simulink model "full_sys_Harness1"  (R2022a)
settings: Solver=FixedStepAuto  StartTime=0.0  StopTime=10.0  RelTol=1e-3  EnableMultiTasking=on
undefined symbols (not defined in the file): sigbuilder_block
settings Model: Creator=FUGAZI  LastModifiedBy=FUGAZI
settings SolverCC: AutoInsertRateTranBlk=on
settings OptimizationCC: EnhancedBackFolding=on  PassReuseOutputArgsAs=Individual arguments  ZeroExternalMemoryAtStartup=off  ZeroInternalMemoryAtStartup=off  MaxStackSize=64  OptimizeBlockOrder=speed  DifferentSizesBufferReuse=on  OptimizationCustomize=off  EfficientTunableParamExpr=on
settings DebuggingCC: ParameterTunabilityLossMsg=error
settings HardwareCC: ProdBitPerPointer=32  ProdBitPerSizeT=32  ProdBitPerPtrDiffT=32  ProdLargestAtomicInteger=Long  ProdLargestAtomicFloat=Double  ProdWordSize=32  ProdLongLongMode=on  ProdHWDeviceType=ARM Compatible->ARM Cortex
settings SFSimCC: MATLABDynamicMemAlloc=off
settings RTWCC: SystemTargetFile=ert.tlc  HardwareBoard=STM32 Nucleo L476RG  TemplateMakefile=ert_default_tmf  Toolchain=GNU Tools for ARM Embedded Processors
settings CodeAppCC: ForceParamTrailComments=on  IgnoreCustomStorageClasses=off  OperatorAnnotations=on  SimulinkDataObjDesc=on  SFDataObjDesc=on  InsertBlockDesc=on
settings ERTTargetCC: ExtModeTransport=3  ExtModeStaticAlloc=on  ExtModeStaticAllocSize=2000  ExtModeMexFile=ext_xcp  ExtModeIntrfLevel=Level2 - Open

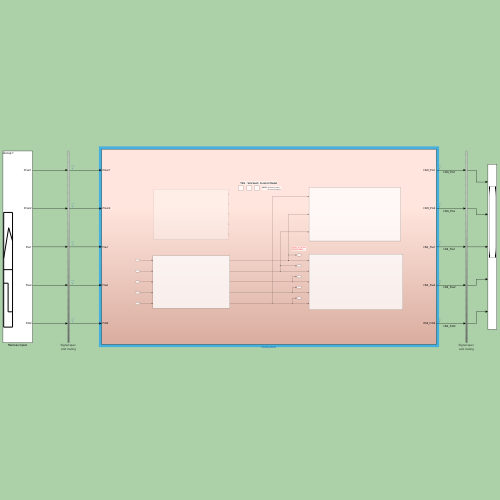
[thumbnail: Simulink's stored preview of the top-level diagram]
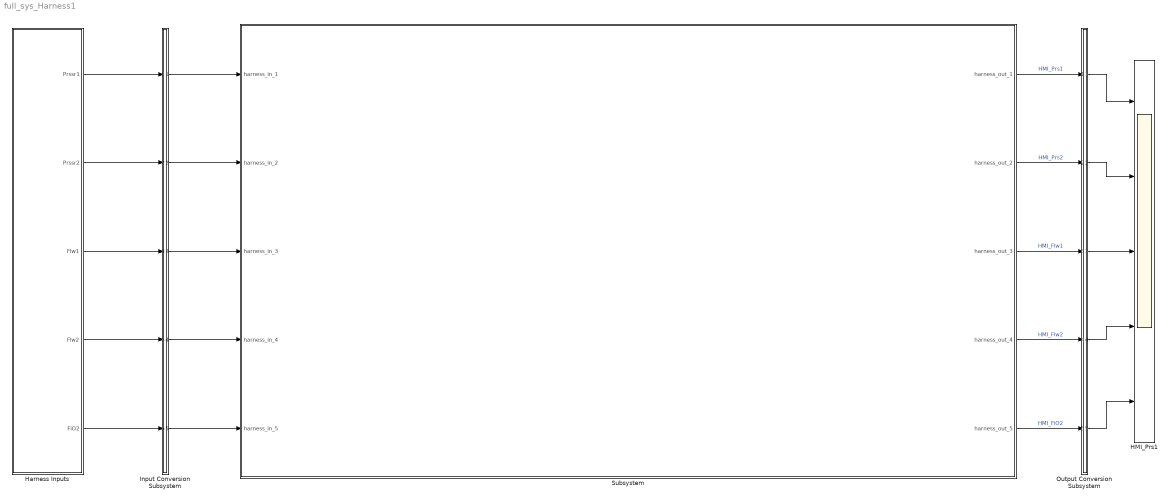
== system full_sys_Harness1 ==
  HMI_Prs1 : Scope
  Harness Inputs : Subsystem  Tag=STV Subsys  LoadFcn=sigbuilder_block('load');  StartFcn=sigbuilder_block('start');  StopFcn=sigbuilder_block('stop');  ClipboardFcn=sigbuilder_block('clipboard');  mask(Sigbuilder block){tuvar=[0:10]}
      mask init:
      | if ~strcmp(get_param(bdroot(gcb),'SimulationStatus'),'stopped'),tuvar = sigbuilder_block('maskInit'); end
      settings: CopyFcn=sigbuilder_block('copy');  DeleteFcn=sigbuilder_block('delete');  ModelCloseFcn=sigbuilder_block('modelClose');  PreSaveFcn=sigbuilder_block('preSave');  PauseFcn=sigbuilder_block('pause');  ContinueFcn=sigbuilder_block('continue');  NameChangeFcn=sigbuilder_block('namechange');  OpenFcn=sigbuilder_block('open',[127.2 33.6 1012.8 503.4 ]);  CloseFcn=sigbuilder_block('close');
      mask Display: plot(0, 0, 100, 100,[2, 2, 32, 32, 2], [68, 8, 8, 68, 68],[32, 2], [38, 38], [32, 19, 2],[53, 60, 44], [32, 17, 17, 2],[16, 16, 31, 31]);txt = getActiveGroup(gcbh);text(2, 100, txt,'verticalAlignment', 'top');
  Input Conversion Subsystem : Subsystem  Tag=__SLT_ICS__  Description=|
      | Signal spec.
      | and routing
      settings: AttributesFormatString=%<Description>
  Output Conversion Subsystem : Subsystem  Tag=__SLT_OCS__  Description=|
      | Signal spec.
      | and routing
      settings: AttributesFormatString=%<Description>
  Subsystem : Subsystem  Tag=__SL_testing_harness_stub_
  wires:
  Harness Inputs/1(Prssr1) -> Input Conversion Subsystem/1(Inport_1)
  Harness Inputs/2(Prssr2) -> Input Conversion Subsystem/2(Inport_2)
  Harness Inputs/3(Flw1) -> Input Conversion Subsystem/3(Inport_3)
  Harness Inputs/4(Flw2) -> Input Conversion Subsystem/4(Inport_4)
  Harness Inputs/5(FiO2) -> Input Conversion Subsystem/5(Inport_5)
  Output Conversion Subsystem/1(Outport_1) -> HMI_Prs1/1
  Output Conversion Subsystem/2(Outport_2) -> HMI_Prs1/2
  Output Conversion Subsystem/3(Outport_3) -> HMI_Prs1/3
  Output Conversion Subsystem/4(Outport_4) -> HMI_Prs1/4
  Output Conversion Subsystem/5(Outport_5) -> HMI_Prs1/5
  Input Conversion Subsystem/1(Outport_1) -> Subsystem/1(harness_in_1)
  Input Conversion Subsystem/2(Outport_2) -> Subsystem/2(harness_in_2)
  Input Conversion Subsystem/3(Outport_3) -> Subsystem/3(harness_in_3)
  Input Conversion Subsystem/4(Outport_4) -> Subsystem/4(harness_in_4)
  Input Conversion Subsystem/5(Outport_5) -> Subsystem/5(harness_in_5)
  Subsystem/1(harness_out_1) -> Output Conversion Subsystem/1(Inport_1)  "HMI_Prs1"
  Subsystem/2(harness_out_2) -> Output Conversion Subsystem/2(Inport_2)  "HMI_Prs2"
  Subsystem/3(harness_out_3) -> Output Conversion Subsystem/3(Inport_3)  "HMI_Flw1"
  Subsystem/4(harness_out_4) -> Output Conversion Subsystem/4(Inport_4)  "HMI_Flw2"
  Subsystem/5(harness_out_5) -> Output Conversion Subsystem/5(Inport_5)  "HMI_FiO2"

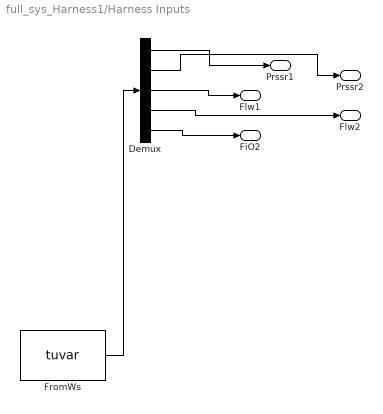
== system full_sys_Harness1/Harness Inputs ==
  Demux : Demux  Tag=STV Demux  Outputs=5
  FromWs : FromWorkspace  Tag=STV FromWs  VariableName=tuvar
      SigBuilderData=|
      | dataSet.timeRange = [0 20]
      | dataSet.name = 'Group 1'
      | sbobj.Name = 'Signal Builder'
      | sbobj.Groups.Name = 'Group 1'
      | sbobj.Groups.Signals(1).Name = 'Prssr1'
      | sbobj.Groups.Signals(1).XData = [0 0.099 2 2 4 4 6 6 8 8 10 10 12 12 14 14 16 16 18 18 20]
      | sbobj.Groups.Signals(1).YData = [0 0 0 6 6 16 16 5 5 18 18 8 8 15 15 4.5 4.5 19 19 0 0]
      | sbobj.Groups.Signals(2).Name = 'Prssr2'
      | sbobj.Groups.Signals(2).XData = [0 2 2 4 4 6 6 7.98 7.98 9.98 9.98 12 12 20]
      | sbobj.Groups.Signals(2).YData = [0 0 5.5 5.5 15 15 6 6 18 18 5 5 0 0]
      | sbobj.Groups.Signals(3).Name = 'Flw1'
      | sbobj.Groups.Signals(3).XData = [0 20]
      | sbobj.Groups.Signals(3).YData = [0 0]
      | sbobj.Groups.Signals(4).Name = 'Flw2'
      | sbobj.Groups.Signals(4).XData = [0 20]
      | sbobj.Groups.Signals(4).YData = [0 0]
      | sbobj.Groups.Signals(5).Name = 'FiO2'
      | sbobj.Groups.Signals(5).XData = [0 20]
      | sbobj.Groups.Signals(5).YData = [0 0]
      | sbobj.Groups.TimeRange = [0 20]
  Prssr1 : Outport  Tag=STV Outport
  Prssr2 : Outport  Tag=STV Outport  Port=2
  Flw1 : Outport  Tag=STV Outport  Port=3
  Flw2 : Outport  Tag=STV Outport  Port=4
  FiO2 : Outport  Tag=STV Outport  Port=5
  wires:
  FromWs/1 -> Demux/1
  Demux/1 -> Prssr1/1
  Demux/2 -> Prssr2/1
  Demux/3 -> Flw1/1
  Demux/4 -> Flw2/1
  Demux/5 -> FiO2/1

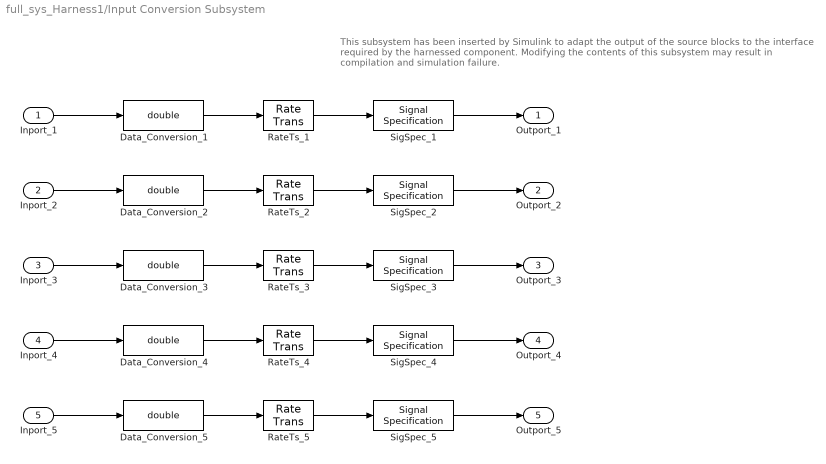
== system full_sys_Harness1/Input Conversion Subsystem ==
  note: This subsystem has been inserted by Simulink to adapt the output of the source blocks to the interface required by the harnessed component.
      |  Modifying the contents of this subsystem may result in compilation and simulation failure.
  Inport_1 : Inport
  Inport_2 : Inport  Port=2
  Inport_3 : Inport  Port=3
  Inport_4 : Inport  Port=4
  Inport_5 : Inport  Port=5
  Data_Conversion_{1..5} (5 alike) : DataTypeConversion  OutDataTypeStr=double
  RateTs_{1..5} (5 alike) : RateTransition  OutPortSampleTime=[-1, 0]
  SigSpec_{1..5} (5 alike) : SignalSpecification  OutDataTypeStr=double  Dimensions=[1]  SampleTime=[-1, 0]
  Outport_1 : Outport
  Outport_2 : Outport  Port=2
  Outport_3 : Outport  Port=3
  Outport_4 : Outport  Port=4
  Outport_5 : Outport  Port=5
  wires:
  SigSpec_1/1 -> Outport_1/1
  RateTs_1/1 -> SigSpec_1/1
  Data_Conversion_1/1 -> RateTs_1/1
  Inport_1/1 -> Data_Conversion_1/1
  SigSpec_2/1 -> Outport_2/1
  RateTs_2/1 -> SigSpec_2/1
  Data_Conversion_2/1 -> RateTs_2/1
  Inport_2/1 -> Data_Conversion_2/1
  SigSpec_3/1 -> Outport_3/1
  RateTs_3/1 -> SigSpec_3/1
  Data_Conversion_3/1 -> RateTs_3/1
  Inport_3/1 -> Data_Conversion_3/1
  SigSpec_4/1 -> Outport_4/1
  RateTs_4/1 -> SigSpec_4/1
  Data_Conversion_4/1 -> RateTs_4/1
  Inport_4/1 -> Data_Conversion_4/1
  SigSpec_5/1 -> Outport_5/1
  RateTs_5/1 -> SigSpec_5/1
  Data_Conversion_5/1 -> RateTs_5/1
  Inport_5/1 -> Data_Conversion_5/1

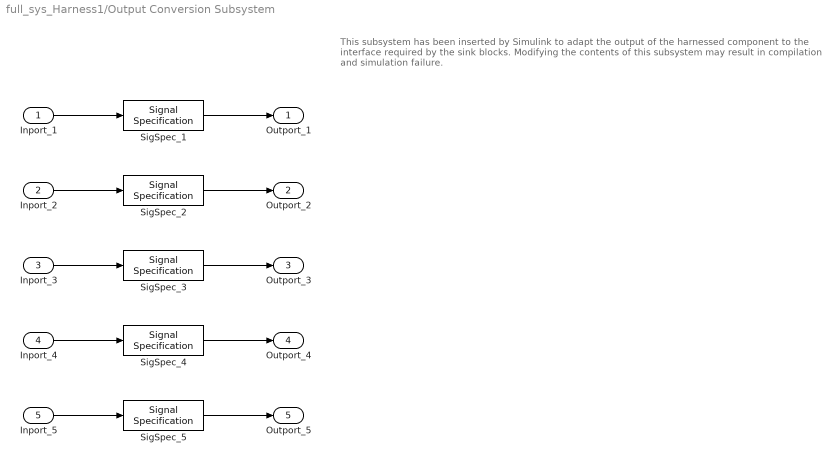
== system full_sys_Harness1/Output Conversion Subsystem ==
  note: This subsystem has been inserted by Simulink to adapt the output of the harnessed component to the interface required by the sink blocks.
      |  Modifying the contents of this subsystem may result in compilation and simulation failure.
  Inport_1 : Inport
  Inport_2 : Inport  Port=2
  Inport_3 : Inport  Port=3
  Inport_4 : Inport  Port=4
  Inport_5 : Inport  Port=5
  SigSpec_{1..5} (5 alike) : SignalSpecification  OutDataTypeStr=double  Dimensions=[1]
  Outport_1 : Outport
  Outport_2 : Outport  Port=2
  Outport_3 : Outport  Port=3
  Outport_4 : Outport  Port=4
  Outport_5 : Outport  Port=5
  wires:
  Inport_1/1 -> SigSpec_1/1
  SigSpec_1/1 -> Outport_1/1
  Inport_2/1 -> SigSpec_2/1
  SigSpec_2/1 -> Outport_2/1
  Inport_3/1 -> SigSpec_3/1
  SigSpec_3/1 -> Outport_3/1
  Inport_4/1 -> SigSpec_4/1
  SigSpec_4/1 -> Outport_4/1
  Inport_5/1 -> SigSpec_5/1
  SigSpec_5/1 -> Outport_5/1

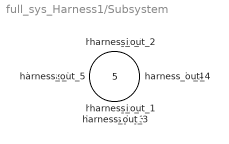
== system full_sys_Harness1/Subsystem ==
  harness_in_1 : Inport
  harness_in_2 : Inport  Port=2
  harness_in_3 : Inport  Port=3
  harness_in_4 : Inport  Port=4
  harness_in_5 : Inport  Port=5
  harness_out_1 : Outport
  harness_out_2 : Outport  Port=2
  harness_out_3 : Outport  Port=3
  harness_out_4 : Outport  Port=4
  harness_out_5 : Outport  Port=5
